simulink model "Exp2_19EE10039_Mansi_PartB"  (R2021a)
settings: Solver=VariableStepAuto  StartTime=0.0  StopTime=0.005  RelTol=1e-3
libraries: spsSeriesRLCBranchLib x5, spsVoltageMeasurementLib x4, spsCurrentMeasurementLib x3, spsDiodeLib x2, spsDCVoltageSourceLib x1, spsLinearTransformerLib x1, spsMeanLib x1, spsMosfetLib x1, spsMultimeterLib x1, spspowerguiLib x1
settings Model: Creator=mansi  LastModifiedBy=mansi

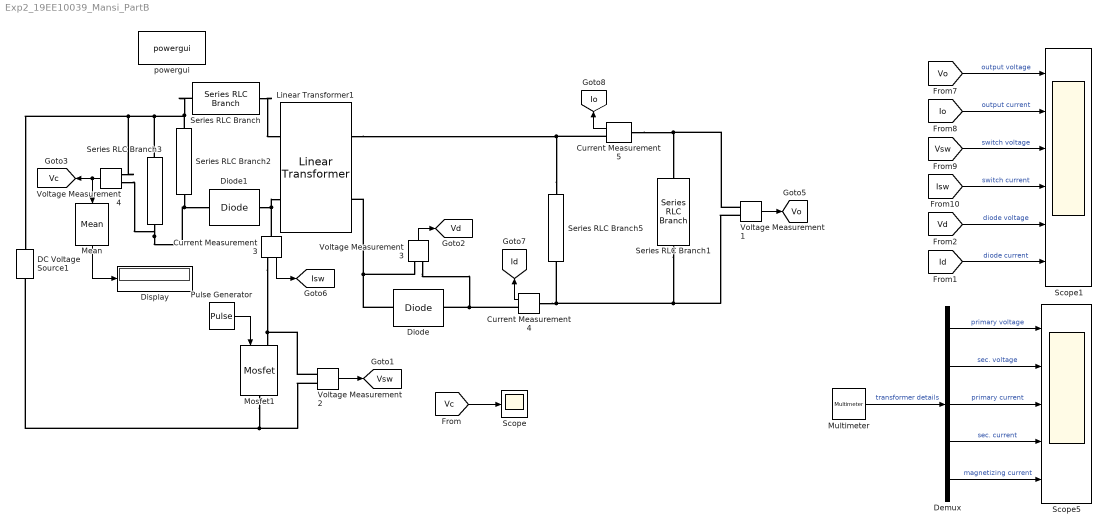
== system Exp2_19EE10039_Mansi_PartB ==
  Current Measurement3 : spsCurrentMeasurementLib/Current Measurement  PhasorSimulation=off  OutputType=Complex  PSBequivalent=0
  Current Measurement4 : spsCurrentMeasurementLib/Current Measurement  PhasorSimulation=off  OutputType=Complex  PSBequivalent=0
  Current Measurement5 : spsCurrentMeasurementLib/Current Measurement  PhasorSimulation=off  OutputType=Complex  PSBequivalent=0
  DC Voltage Source1 : spsDCVoltageSourceLib/DC Voltage Source  Amplitude=24  Measurements=None
  Demux : Demux  Outputs=5
  Diode : spsDiodeLib/Diode  Ron=1e-6  Lon=0  Vf=0  IC=0  UseSnubber=0  Rs=inf  Cs=0  Measurements=off
  Diode1 : spsDiodeLib/Diode  Ron=1e-6  Lon=0  Vf=0  IC=0  UseSnubber=0  Rs=inf  Cs=0  Measurements=off
  Display : Display
  Linear Transformer1 : spsLinearTransformerLib/Linear Transformer  UNITS=SI  NominalPower=[20 100000 ]  winding1=[30 0 0]  winding2=[10 0 0]  ThreeWindings=off  winding3=[3.15e+05 0.7938 0.084225]  RmLm=[1e12 250e-6]  Measurements=All voltages and currents  DataType=on
  Mean : spsMeanLib/Mean  Freq=100000  Vinit=0  Ts=0
  Mosfet1 : spsMosfetLib/Mosfet  Ron=1e-6  Lon=0  Rd=1e-6  Vfd=0  IC=0  Rs=1e12  Cs=inf  Measurements=off
  Multimeter : spsMultimeterLib/Multimeter  PhasorSimulation=off  OutputType=Complex  sel=[1 2 3 4 6]  L=7  Gain=[1 1 1 1 1]  yselected={'Uw1: Linear Transformer1','Uw2: Linear Transformer1','Iw1: Linear Transformer1','Iw2: Linear Transformer1','Imag: Linear Transformer1'};  PSBOutputType=1  PSBequivalent=0  AxesSetting=[0,0.1,-100,100]  Display=0  SavedBlockNames=-11
  Pulse Generator : DiscretePulseGenerator  PulseType=Time based  Period=1/100000  PulseWidth=40
  Scope : Scope
  Scope1 : Scope  NumInputPorts=6
  Scope5 : Scope  NumInputPorts=5
  Series RLC Branch : spsSeriesRLCBranchLib/Series RLC Branch  LConnTagsString=__new0  RConnTagsString=__new0  BranchType=L  Resistance=1  Inductance=450e-9  SetiL0=off  InitialCurrent=0  Capacitance=1e-6  Setx0=off  InitialVoltage=0  Measurements=None
  Series RLC Branch1 : spsSeriesRLCBranchLib/Series RLC Branch  LConnTagsString=__new0  RConnTagsString=__new0  BranchType=R  Resistance=1  Inductance=1e-3  SetiL0=off  InitialCurrent=0  Capacitance=1e-6  Setx0=off  InitialVoltage=0  Measurements=None
  Series RLC Branch2 : spsSeriesRLCBranchLib/Series RLC Branch  LConnTagsString=__new0  RConnTagsString=__new0  BranchType=R  Resistance=5000  Inductance=1e-3  SetiL0=off  InitialCurrent=0  Capacitance=100e-6  Setx0=off  InitialVoltage=0  Measurements=None
  Series RLC Branch3 : spsSeriesRLCBranchLib/Series RLC Branch  LConnTagsString=__new0  RConnTagsString=__new0  BranchType=C  Resistance=0  Inductance=1e-3  SetiL0=off  InitialCurrent=0  Capacitance=10e-9  Setx0=off  InitialVoltage=0  Measurements=None
  Series RLC Branch5 : spsSeriesRLCBranchLib/Series RLC Branch  LConnTagsString=__new0  RConnTagsString=__new0  BranchType=C  Resistance=0  Inductance=1e-3  SetiL0=off  InitialCurrent=0  Capacitance=100e-6  Setx0=off  InitialVoltage=0  Measurements=None
  Voltage Measurement{1..4} (4 alike) : spsVoltageMeasurementLib/Voltage Measurement  PhasorSimulation=off  OutputType=Complex  PSBequivalent=0
  powergui : spspowerguiLib/powergui  Priority=1  SimulationMode=Discrete  SampleTime=1e-7  frequency=60  Iterations=50  frequencyindice=0  Pbase=100e6  ErrMax=1e-4  UnitsV=kV  UnitsW=MW  buscounter=0  FunctionMessages=off  echomessages=off  EnableUseOfTLC=off  CurrentSourceSwitches=off  DisableSnubberDevices=off  DisableRonSwitches=off  DisableVfSwitches=off  DisplayEquations=off  AutomaticDiscreteSolvers=off  SolverType=Tustin/Backward Euler (TBE)  Interpol=off  ExternalGateDelay=off  methode=off  Ts=100  x0status=blocks  SPID=on  SwTol=0  HookPort=off  NonlinearTolerance=1e-4  nMaxIteration=100  ContinueOnMaxIteration=off  RestoreLinks=warning  ResistiveCurrentMeasurement=off  Frange=[0:2:500]  Ylog=off  Xlog=on  ShowGrid=off  save=off  variable=ZData  structure=0  ZoomFFT=off  StartTime=0.0  cycles=1  DisplayStyle=1  fundamental=60  FreqAxis=off  MaxFrequency=1000  frequencyindicesteady=1  RmsSteady=1  display=off
  tag scope: Id=global, Io=global, Isw=global, Vc=global, Vd=global, Vo=global, Vsw=global
  wires:
  Demux/4 -> Scope5/4  "sec. current"
  [Vd] -> Scope1/5  "diode voltage"
  [Vo] -> Scope1/1  "output voltage"
  Demux/5 -> Scope5/5  "magnetizing current"
  Current Measurement3/1 -> [Isw]
  Mean/1 -> Display/1
  Demux/2 -> Scope5/2  "sec. voltage"
  Current Measurement5/1 -> [Io]
  [Vsw] -> Scope1/3  "switch voltage"
  [Isw] -> Scope1/4  "switch current"
  Current Measurement4/1 -> [Id]
  Voltage Measurement3/1 -> [Vd]
  Multimeter/1 -> Demux/1  "transformer details"
  Voltage Measurement2/1 -> [Vsw]
  Voltage Measurement4/1 -> Mean/1, [Vc]
  [Id] -> Scope1/6  "diode current"
  Demux/3 -> Scope5/3  "primary current"
  [Io] -> Scope1/2  "output current"
  Demux/1 -> Scope5/1  "primary voltage"
  [Vc] -> Scope/1
  Pulse Generator/1 -> Mosfet1/1
  Voltage Measurement1/1 -> [Vo]
  connections:
  Voltage Measurement1/LConn1 -- Series RLC Branch1/LConn1 -- Current Measurement4/LConn1 -- Series RLC Branch5/LConn1
  Voltage Measurement2/LConn1 -- Mosfet1/LConn1 -- Current Measurement3/RConn1
  DC Voltage Source1/LConn1 -- Voltage Measurement2/LConn2 -- Mosfet1/RConn1
  Series RLC Branch5/RConn1 -- Current Measurement5/RConn1 -- Linear Transformer1/RConn1
  Diode/RConn1 -- Voltage Measurement3/LConn2 -- Current Measurement4/RConn1
  Diode1/LConn1 -- Current Measurement3/LConn1 -- Linear Transformer1/LConn2
  Series RLC Branch/LConn1 -- Series RLC Branch2/RConn1 -- Voltage Measurement4/LConn2 -- DC Voltage Source1/RConn1 -- Series RLC Branch3/RConn1
  Series RLC Branch2/LConn1 -- Series RLC Branch3/LConn1 -- Voltage Measurement4/LConn1 -- Diode1/RConn1
  Current Measurement5/LConn1 -- Series RLC Branch1/RConn1 -- Voltage Measurement1/LConn2
  Voltage Measurement3/LConn1 -- Linear Transformer1/RConn2 -- Diode/LConn1
  Series RLC Branch/RConn1 -- Linear Transformer1/LConn1
